simulink model "aeroSurface_th"  (R2018b)
settings: Solver=VariableStepAuto  StartTime=0.0  StopTime=0  RelTol=1e-3
values from neighbouring files (symbols this model uses):
  defAng = 0*pi/180    (= 0)    [aeroSurface_ts1.m]    (also in aeroSurface_ts2.m = -0.0174532925199)
  dynPress = 1    [aeroSurface_ts1.m]    (also in aeroSurface_ts2.m)
  uAppBody = uAppBody/sqrt(sum(uAppBody.^2))    [aeroSurface_ts1.m]    (also in aeroSurface_ts2.m)
libraries: aeroSurface_ul x1
settings Model: Creator=mcobb  LastModifiedBy=mcobb

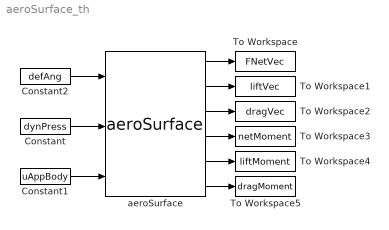
== system aeroSurface_th ==
  Constant : Constant  Value=dynPress
  Constant1 : Constant  Value=uAppBody
  Constant2 : Constant  Value=defAng
  To Workspace : ToWorkspace  VariableName=FNetVec  SaveFormat=Timeseries  SampleTime=-1
  To Workspace1 : ToWorkspace  VariableName=liftVec  SaveFormat=Timeseries  SampleTime=-1
  To Workspace2 : ToWorkspace  VariableName=dragVec  SaveFormat=Timeseries  SampleTime=-1
  To Workspace3 : ToWorkspace  VariableName=netMoment  SaveFormat=Timeseries  SampleTime=-1
  To Workspace4 : ToWorkspace  VariableName=liftMoment  SaveFormat=Timeseries  SampleTime=-1
  To Workspace5 : ToWorkspace  VariableName=dragMoment  SaveFormat=Timeseries  SampleTime=-1
  aeroSurface : aeroSurface_ul/aeroSurface  rAeroCent=aeroCenterVec  uSpan=spanRotationVec  uChord=chordDirectionVec  ClFitParams=ClFitParams  CdFitParams=CdFitParams  ARef=refArea
  wires:
  Constant/1 -> aeroSurface/2
  Constant1/1 -> aeroSurface/3
  aeroSurface/1 -> To Workspace/1
  aeroSurface/6 -> To Workspace5/1
  aeroSurface/5 -> To Workspace4/1
  aeroSurface/4 -> To Workspace3/1
  aeroSurface/3 -> To Workspace2/1
  aeroSurface/2 -> To Workspace1/1
  Constant2/1 -> aeroSurface/1
